simulink model "bai29"  (R2016a)
settings: Solver=VariableStepAuto  StartTime=0.0  StopTime=10.0  RelTol=1e-3
settings Model: Creator=HP  LastModifiedBy=HP

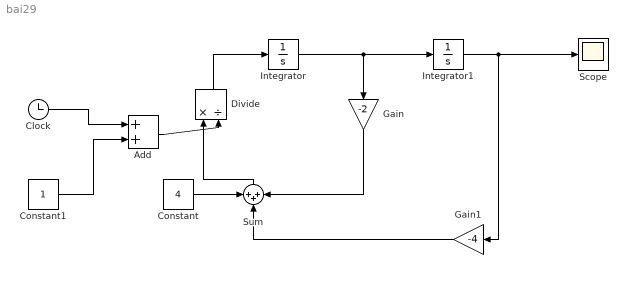
== system bai29 ==
  Add : Sum
  Clock : Clock
  Constant : Constant  Value=4
  Constant1 : Constant
  Divide : Product  Inputs=*/
  Gain : Gain  Gain=-2
  Gain1 : Gain  Gain=-4
  Integrator : Integrator  InitialCondition=1
  Integrator1 : Integrator  InitialCondition=1
  Scope : Scope
  Sum : Sum  Inputs=+++
  wires:
  Integrator/1 -> Gain/1, Integrator1/1
  Integrator1/1 -> Scope/1, Gain1/1
  Gain/1 -> Sum/3
  Gain1/1 -> Sum/2
  Constant/1 -> Sum/1
  Sum/1 -> Divide/1
  Divide/1 -> Integrator/1
  Clock/1 -> Add/1
  Constant1/1 -> Add/2
  Add/1 -> Divide/2
